simulink model "ProjectModel"  (R2025a)
settings: Solver=VariableStepAuto  StartTime=0.0  StopTime=5  RelTol=1e-3
model workspace (MAT data in the model file):
  M = 0.5
  Ts = 0.01
  b = 0.1
  g = 9.8
  l = 0.5
  m = 0.2
settings Model: Creator=sturton  LastModifiedBy=JPIRES3

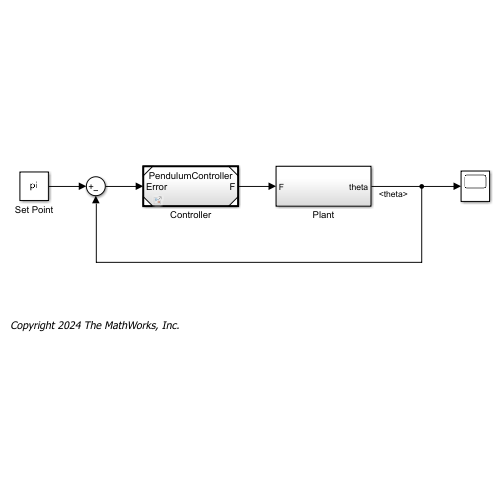
[thumbnail: Simulink's stored preview of the top-level diagram]
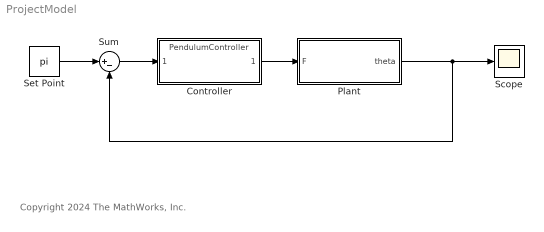
== system ProjectModel ==
  note: Copyright 2024 The MathWorks, Inc.
  Controller : ModelReference  ModelNameDialog=PendulumController.slx  SimulationMode=Normal  ModelReferenceVersion=3.2
  Plant : Subsystem
  Scope : Scope
      settings: ActiveDisplayYMinimum=3.1337618061803703  ActiveDisplayYMaximum=3.199656919982754
  Set Point : Constant  Value=pi
  Sum : Sum  Inputs=|+-
  wires:
  Plant/1(theta) -> Scope/1, Sum/2
  Set Point/1 -> Sum/1
  Sum/1 -> Controller/1
  Controller/1 -> Plant/1(F)

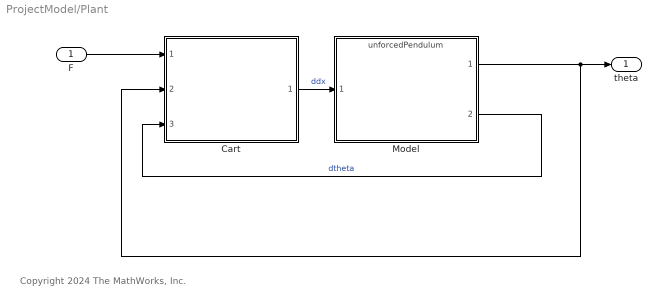
== system ProjectModel/Plant ==
  note: Copyright 2024 The MathWorks, Inc.
  F : Inport
  Cart : Subsystem  ReferencedSubsystem=CartBase
  Model : ModelReference  ModelNameDialog=unforcedPendulum.slx  SimulationMode=Normal  ModelReferenceVersion=1.19
  theta : Outport
  wires:
  F/1 -> Cart/1
  Cart/1 -> Model/1  "ddx"
  Model/2 -> Cart/3  "dtheta"
  Model/1 -> Cart/2, theta/1
